simulink model "PlantModel"  (R2022b)
settings: Solver=VariableStepAuto  StartTime=0.0  StopTime=20  RelTol=1e-3
settings Model: Creator=steph  LastModifiedBy=steph
settings OptimizationCC: BlockReduction=off  DefaultParameterBehavior=Inlined  BufferReuse=off

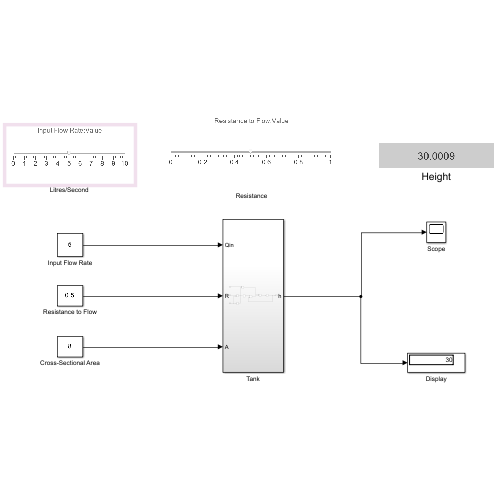
[thumbnail: Simulink's stored preview of the top-level diagram]
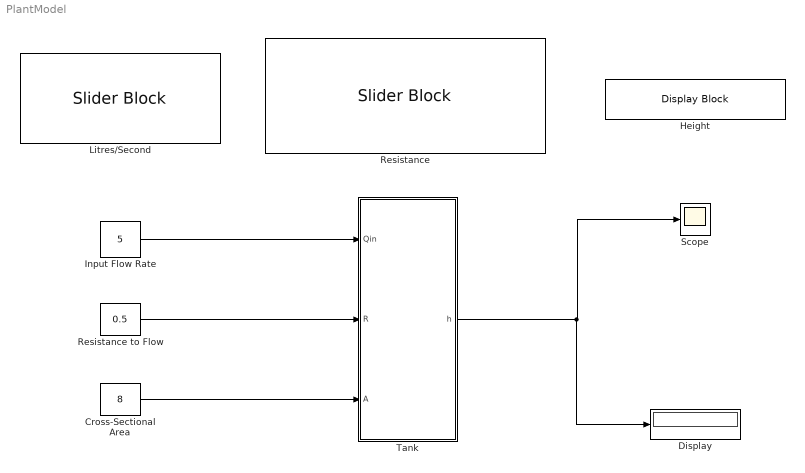
== system PlantModel ==
  Cross-Sectional Area : Constant  Value=8  OutMin=0  OutMax=200
  Display : Display
  Height : DisplayBlock  LabelPosition=Hide  Transparency=1
  Input Flow Rate : Constant  Value=5
  "Litres/Second " : SliderBlock  ScaleMax=10
  Resistance : SliderBlock  ScaleMax=1  TickInterval=0.2
  Resistance to Flow : Constant  Value=0.5  OutMin=0
  Scope : Scope
  Tank : Subsystem
  wires:
  Input Flow Rate/1 -> Tank/1(Qin)
  Resistance to Flow/1 -> Tank/2(R)
  Cross-Sectional Area/1 -> Tank/3(A)
  Tank/1(h) -> Display/1, Scope/1

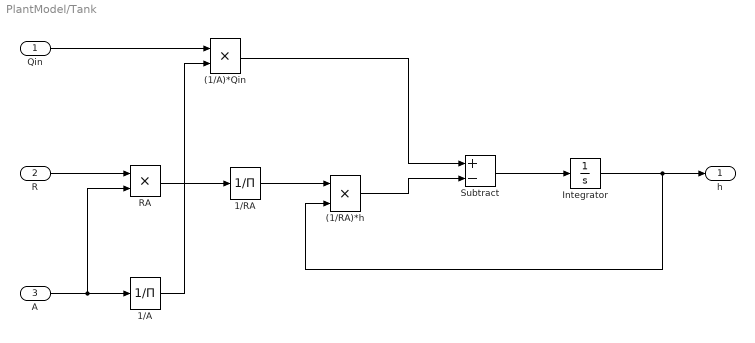
== system PlantModel/Tank ==
  Qin : Inport
  R : Inport  Port=2
  A : Inport  Port=3
  (1/A)*Qin : Product
  (1/RA)*h : Product
  1/A : Product  Inputs=/
  1/RA : Product  Inputs=/
  Integrator : Integrator
  RA : Product
  Subtract : Sum  Inputs=+-
  h : Outport
  wires:
  A/1 -> RA/2, 1/A/1
  R/1 -> RA/1
  RA/1 -> 1/RA/1
  1/A/1 -> (1/A)*Qin/2
  1/RA/1 -> (1/RA)*h/1
  (1/A)*Qin/1 -> Subtract/1
  (1/RA)*h/1 -> Subtract/2
  Integrator/1 -> (1/RA)*h/2, h/1
  Qin/1 -> (1/A)*Qin/1
  Subtract/1 -> Integrator/1
